simulink library "rocket_thrust_data_library"  (R2014a)
settings: Solver=ode45  StartTime=0.0  StopTime=10.0  RelTol=1e-3
settings Model: Creator=scorpii  LastModifiedBy=scorpii

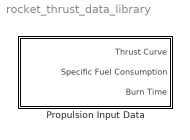
== system rocket_thrust_data_library ==
  Propulsion Input Data : Subsystem

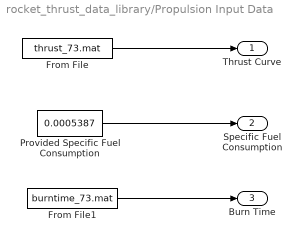
== system rocket_thrust_data_library/Propulsion Input Data ==
  From File : FromFile  FileName=thrust_73.mat  OutDataTypeStr=double  ExtrapolationBeforeFirstDataPoint=Hold first value  InterpolationWithinTimeRange=Zero order hold  ExtrapolationAfterLastDataPoint=Hold last value
  From File1 : FromFile  FileName=burntime_73.mat  SampleTime=0
  Provided Specific Fuel Consumption : Constant  Value=0.0005387
  Thrust Curve : Outport
  Specific Fuel Consumption : Outport  Port=2
  Burn Time : Outport  Port=3
  wires:
  Provided Specific Fuel Consumption/1 -> Specific Fuel Consumption/1
  From File1/1 -> Burn Time/1
  From File/1 -> Thrust Curve/1
